simulink model "DC_PID"  (R2015a)
settings: Solver=ode45  StartTime=0.0  StopTime=50.0  RelTol=1e-3
values from neighbouring files (symbols this model uses):
  J = 10    [DC_PID_IMC.m]    (also in DCtest.m; data.mat)
  KE = 8.50    (= 8.5)    [DC_PID_IMC.m]    (also in DCtest.m; data.mat)
  Kp = 0.1764    [DC_PID_IMC.m]    (also in DCtest.m; data.mat)
  KT = 8.50    (= 8.5)    [DC_PID_IMC.m]    (also in DCtest.m; data.mat)
  La = 0.003    [DC_PID_IMC.m]    (also in DCtest.m; data.mat)
  Ra = 0.15    [DC_PID_IMC.m]    (also in DCtest.m; data.mat)
  Td = 0.0200    (= 0.02)    [DC_PID_IMC.m]    (also in DCtest.m; data.mat)
  Ti = 0.0208    [DC_PID_IMC.m]    (also in DCtest.m; data.mat)
  TL = 0    [DC_PID_IMC.m]    (also in DCtest.m; data.mat)
settings Model: Creator=yusuke  LastModifiedBy=yusuke

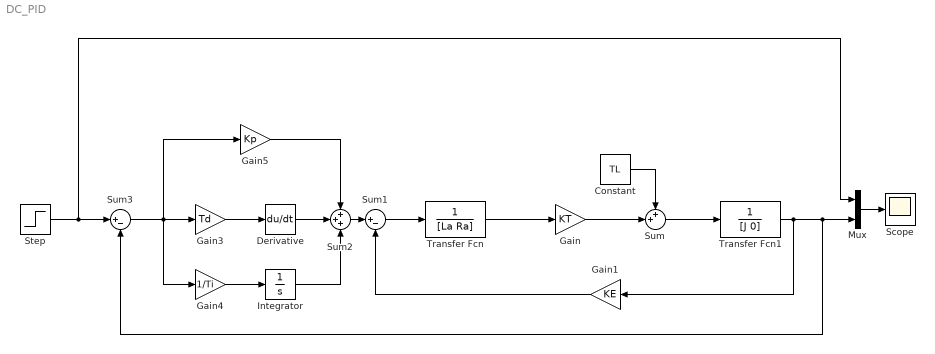
== system DC_PID ==
  Constant : Constant  Value=TL
  Derivative : Derivative
  Gain : Gain  Gain=KT
  Gain1 : Gain  Gain=KE
  Gain3 : Gain  Gain=Td
  Gain4 : Gain  Gain=1/Ti
  Gain5 : Gain  Gain=Kp
  Integrator : Integrator
  Mux : Mux  Inputs=2
  Scope : Scope
      settings: TimeRange=2  YMin=-1.080841638981175  YMax=2.919158361018825
  Step : Step  Time=0  After=100  SampleTime=0
  Sum : Sum  Inputs=++|
  Sum1 : Sum  Inputs=|+-
  Sum2 : Sum  Inputs=+++
  Sum3 : Sum  Inputs=|+-
  Transfer Fcn : TransferFcn  Denominator=[La Ra]
  Transfer Fcn1 : TransferFcn  Denominator=[J 0]
  wires:
  Transfer Fcn/1 -> Gain/1
  Gain/1 -> Sum/2
  Constant/1 -> Sum/1
  Sum/1 -> Transfer Fcn1/1
  Transfer Fcn1/1 -> Sum3/2, Mux/2, Gain1/1
  Gain1/1 -> Sum1/2
  Sum1/1 -> Transfer Fcn/1
  Step/1 -> Sum3/1, Mux/1
  Mux/1 -> Scope/1
  Sum2/1 -> Sum1/1
  Derivative/1 -> Sum2/2
  Gain5/1 -> Sum2/1
  Integrator/1 -> Sum2/3
  Gain3/1 -> Derivative/1
  Gain4/1 -> Integrator/1
  Sum3/1 -> Gain4/1, Gain3/1, Gain5/1
